simulink model "PID"  (R2022b)
settings: Solver=VariableStepAuto  StartTime=0.0  StopTime=10.0  RelTol=1e-3
undefined symbols (not defined in the file): Kd, Ki, Kp, Kw
settings Model: Creator=emanuelevitetta  LastModifiedBy=emanuelevitetta

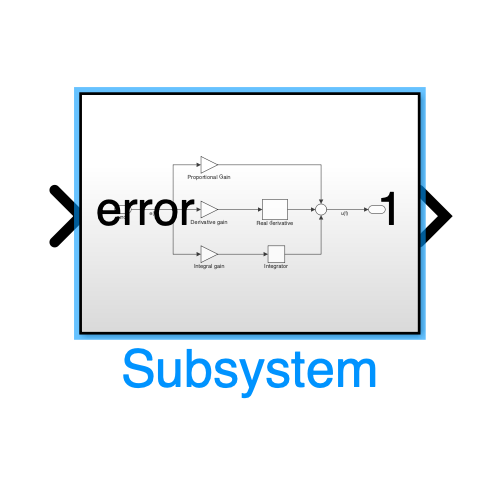
[thumbnail: Simulink's stored preview of the top-level diagram]
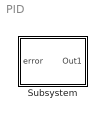
== system PID ==
  Subsystem : Subsystem

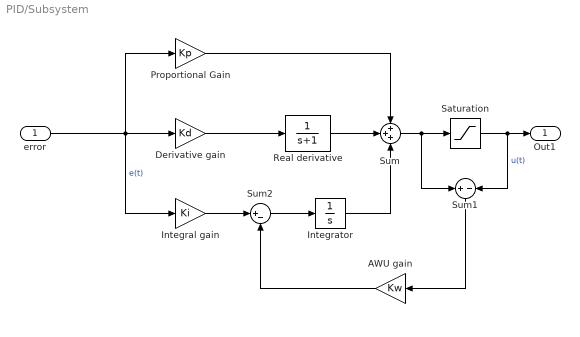
== system PID/Subsystem ==
  error : Inport
  AWU gain : Gain  Gain=Kw
  Derivative gain : Gain  Gain=Kd
  Integral gain : Gain  Gain=Ki
  Integrator : Integrator
  Proportional Gain : Gain  Gain=Kp
  Real derivative : TransferFcn  Denominator=[1 1]
  Saturation : Saturate
  Sum : Sum  Inputs=+++
  Sum1 : Sum  Inputs=+-
  Sum2 : Sum  Inputs=|+-
  Out1 : Outport
  wires:
  Sum/1 -> Sum1/1, Saturation/1
  Proportional Gain/1 -> Sum/1
  Derivative gain/1 -> Real derivative/1
  error/1 -> Integral gain/1, Proportional Gain/1, Derivative gain/1  "e(t)"
  Integrator/1 -> Sum/3
  Real derivative/1 -> Sum/2
  Saturation/1 -> Sum1/2, Out1/1  "u(t)"
  Integral gain/1 -> Sum2/1
  Sum2/1 -> Integrator/1
  AWU gain/1 -> Sum2/2
  Sum1/1 -> AWU gain/1
